simulink model "Traj"  (R2024b)
settings: Solver=VariableStepAuto  StartTime=0.0  StopTime=40  RelTol=1e-3
values from neighbouring files (symbols this model uses):
  K = lqr(A, B, Q, R)    [lq.m]    (also in lqr.m = lqr(A,B,Q,R))
  L = 0.4    [lq.m]    (also in lqr.m = 0.2)
  P = double(P)    [lq.m]    (also in lqr.m)
  theta0 = double(theta0)    [lq.m]    (also in lqr.m)
  theta_ref = double(theta_ref(:))    [lq.m]    (also in lqr.m)
  Ts_ref = double(Ts_ref)    [lq.m]    (also in lqr.m)
  vd_ref = double(vd_ref(:))    [lq.m]    (also in lqr.m)
  wd_ref = double(wd_ref(:))    [lq.m]    (also in lqr.m)
  x0 = double(x0)    [lq.m]    (also in lqr.m)
  y0 = double(y0)    [lq.m]    (also in lqr.m)
libraries: eeGeneralControl x2, slpidlib x2
settings Model: Creator=mwali  LastModifiedBy=mwali
settings ConfigComp: CovBoundaryAbsTol=1.0e-5

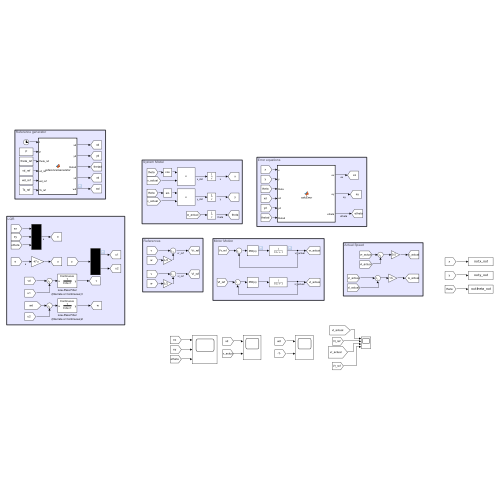
[thumbnail: Simulink's stored preview of the top-level diagram]
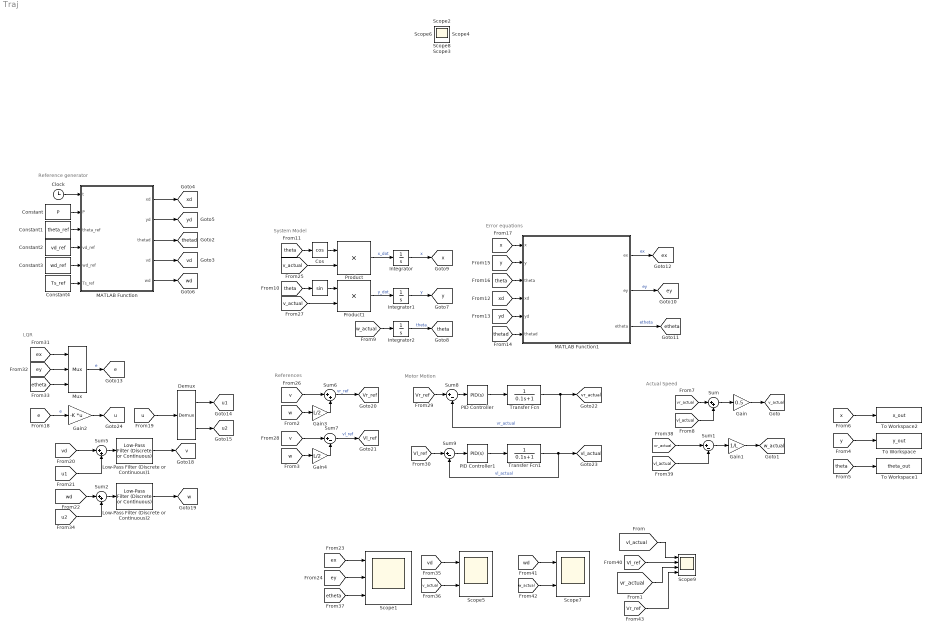
== system Traj ==
  note: Actual Speed
  note: Motor Motion
  note: References
  note: LQR
  note: Error equations
  note: System Model
  note: Reference generator
  " " : Trigonometry
  Clock : Clock
  Constant : Constant  Value=P
  Constant1 : Constant  Value=theta_ref
  Constant2 : Constant  Value=vd_ref
  Constant3 : Constant  Value=wd_ref
  Constant4 : Constant  Value=Ts_ref
  Cos : Trigonometry  Operator=cos
  Demux : Demux  Outputs=2
  Gain : Gain  Gain=0.5
  Gain1 : Gain  Gain=1/L
  Gain2 : Gain  Gain=-K  Multiplication=Matrix(K*u)
  Gain3 : Gain  Gain=L/2
  Gain4 : Gain  Gain=L/2
  Integrator : Integrator  InitialCondition=x0
  Integrator1 : Integrator  InitialCondition=y0
  Integrator2 : Integrator  InitialCondition=theta0
  Low-Pass Filter (Discrete or Continuous)1 : eeGeneralControl/Low-Pass Filter (Discrete or Continuous)  K=1  T=0.6  B=inf  A=-inf  init_option=Inherited from block input  x0=0  Ts=0
  Low-Pass Filter (Discrete or Continuous)2 : eeGeneralControl/Low-Pass Filter (Discrete or Continuous)  K=1  T=0.6  B=inf  A=-inf  init_option=Inherited from block input  x0=0  Ts=0
  MATLAB Function : MATLAB Function  TreatAsAtomicUnit=on
  MATLAB Function1 : MATLAB Function  TreatAsAtomicUnit=on
  Mux : Mux  Inputs=3
  PID Controller : slpidlib/PID Controller  Controller=PID  Form=Parallel  TimeDomain=Continuous-time  UseExternalTs=off  SampleTime=-1  IntegratorMethod=Forward Euler  FilterMethod=Forward Euler  ControllerParametersSource=internal  P=0.9  I=0.04  UseKiTs=off  D=1  UseExternalDerivativeSource=off  N=100  UseFilter=on  TunerSelectOption=Transfer Function Based (PID Tuner App)  InitialConditionSource=internal  InitialConditionForIntegrator=0  InitialConditionForFilter=0  DifferentiatorICPrevScaledInput=0  ExternalReset=none  TrackingMode=off  Kt=1  LimitOutput=off  SatLimitsSource=internal  UpperSaturationLimit=0.5  LowerSaturationLimit=0  LinearizeAsGain=on  AntiWindupMode=clamping  Kb=1  LimitIntegrator=off  UpperIntegratorSaturationLimit=inf  LowerIntegratorSaturationLimit=-inf  POutMin=[]  POutMax=[]  IOutMin=[]  IOutMax=[]  DOutMin=[]  DOutMax=[]  NOutMin=[]  NOutMax=[]  SumOutMin=[]  SumOutMax=[]  SaturationOutMin=[]  SaturationOutMax=[]  PParamMin=[]  PParamMax=[]  IParamMin=[]  IParamMax=[]  DParamMin=[]  DParamMax=[]  NParamMin=[]  NParamMax=[]  KbParamMin=[]  KbParamMax=[]  KtParamMin=[]  KtParamMax=[]  KbOutMin=[]  KbOutMax=[]  KtOutMin=[]  KtOutMax=[]  IntegratorOutMin=[]  IntegratorOutMax=[]  FilterOutMin=[]  FilterOutMax=[]  SumI1OutMin=[]  SumI1OutMax=[]  SumI2OutMin=[]  SumI2OutMax=[]  SumI3OutMin=[]  SumI3OutMax=[]  SumI4OutMin=[]  SumI4OutMax=[]  SumDOutMin=[]  SumDOutMax=[]  DifferentiatorOutMin=[]  DifferentiatorOutMax=[]  FilterDiffOutCoefMin=[]  FilterDiffOutCoefMax=[]  ReciprocalOutMin=[]  ReciprocalOutMax=[]  SumDenOutMin=[]  SumDenOutMax=[]  SumNumOutMin=[]  SumNumOutMax=[]  DivideOutMin=[]  DivideOutMax=[]  UdiffTsProdOutMin=[]  UdiffTsProdOutMax=[]  NTsProdOutMin=[]  NTsProdOutMax=[]  UintegralTsProdOutMin=[]  UintegralTsProdOutMax=[]  UngainTsProdOutMin=[]  UngainTsProdOutMax=[]  ClampingZeroOutDataTypeStr=Inherit: Inherit via back propagation  ClampingZeroOutMin=[]  ClampingZeroOutMax=[]  FilterDenConstantOutDataTypeStr=Inherit: Inherit via back propagation  FilterDenConstantOutMin=[]  FilterDenConstantOutMax=[]  PCopyOutDataTypeStr=Inherit: Inherit via back propagation  PCopyOutMin=[]  PCopyOutMax=[]  NCopyOutDataTypeStr=Inherit: Inherit via back propagation  NCopyOutMin=[]  NCopyOutMax=[]  IntegratorContinuousStateAttributes=''  IntegratorStateMustResolveToSignalObject=off  IntegratorRTWStateStorageClass=Auto  FilterContinuousStateAttributes=''  FilterStateMustResolveToSignalObject=off  FilterRTWStateStorageClass=Auto  ParallelPVariant=InternalParameters  IdealPVariant=Disabled  IVariant=InternalParameters  DVariant=InternalParameters  IntegratorVariant=Continuous  SatVariant=Disabled  AWVariant=Passthrough  PCopyVariant=Disabled  TRVariant=Disabled  FdbkBlocksVariant=Forward  IdealPFdbkVariant=Disabled  SatFdbkVariant=Disabled  DerivativeFilterVariant=ContFilter  NVariant=InternalParameters  NCopyVariant=Disabled  FilterICVariant=InternalICsFilter  IntegratorICVariant=InternalICs  ExternalResetVariant=Disabled  TRSumVariant=Passthrough  SumFdbkVariant=Disabled  SumVariant=Sum_PID  TsampFilterVariant=InternalTs  TsampNgainVariant=Passthrough  TsampIntegralVariant=Disabled_SignalSpec  ExternalSaturationOutDataTypeStr=Inherit: Same as second input  DerivativeSourceVariant=ErrorSignal  PreIntVariant=InternalPreInt
  PID Controller1 : slpidlib/PID Controller  Controller=PID  Form=Parallel  TimeDomain=Continuous-time  UseExternalTs=off  SampleTime=-1  IntegratorMethod=Forward Euler  FilterMethod=Forward Euler  ControllerParametersSource=internal  P=0.9  I=0.04  UseKiTs=off  D=1  UseExternalDerivativeSource=off  N=100  UseFilter=on  TunerSelectOption=Transfer Function Based (PID Tuner App)  InitialConditionSource=internal  InitialConditionForIntegrator=0  InitialConditionForFilter=0  DifferentiatorICPrevScaledInput=0  ExternalReset=none  TrackingMode=off  Kt=1  LimitOutput=off  SatLimitsSource=internal  UpperSaturationLimit=0.5  LowerSaturationLimit=0  LinearizeAsGain=on  AntiWindupMode=clamping  Kb=1  LimitIntegrator=off  UpperIntegratorSaturationLimit=inf  LowerIntegratorSaturationLimit=-inf  POutMin=[]  POutMax=[]  IOutMin=[]  IOutMax=[]  DOutMin=[]  DOutMax=[]  NOutMin=[]  NOutMax=[]  SumOutMin=[]  SumOutMax=[]  SaturationOutMin=[]  SaturationOutMax=[]  PParamMin=[]  PParamMax=[]  IParamMin=[]  IParamMax=[]  DParamMin=[]  DParamMax=[]  NParamMin=[]  NParamMax=[]  KbParamMin=[]  KbParamMax=[]  KtParamMin=[]  KtParamMax=[]  KbOutMin=[]  KbOutMax=[]  KtOutMin=[]  KtOutMax=[]  IntegratorOutMin=[]  IntegratorOutMax=[]  FilterOutMin=[]  FilterOutMax=[]  SumI1OutMin=[]  SumI1OutMax=[]  SumI2OutMin=[]  SumI2OutMax=[]  SumI3OutMin=[]  SumI3OutMax=[]  SumI4OutMin=[]  SumI4OutMax=[]  SumDOutMin=[]  SumDOutMax=[]  DifferentiatorOutMin=[]  DifferentiatorOutMax=[]  FilterDiffOutCoefMin=[]  FilterDiffOutCoefMax=[]  ReciprocalOutMin=[]  ReciprocalOutMax=[]  SumDenOutMin=[]  SumDenOutMax=[]  SumNumOutMin=[]  SumNumOutMax=[]  DivideOutMin=[]  DivideOutMax=[]  UdiffTsProdOutMin=[]  UdiffTsProdOutMax=[]  NTsProdOutMin=[]  NTsProdOutMax=[]  UintegralTsProdOutMin=[]  UintegralTsProdOutMax=[]  UngainTsProdOutMin=[]  UngainTsProdOutMax=[]  ClampingZeroOutDataTypeStr=Inherit: Inherit via back propagation  ClampingZeroOutMin=[]  ClampingZeroOutMax=[]  FilterDenConstantOutDataTypeStr=Inherit: Inherit via back propagation  FilterDenConstantOutMin=[]  FilterDenConstantOutMax=[]  PCopyOutDataTypeStr=Inherit: Inherit via back propagation  PCopyOutMin=[]  PCopyOutMax=[]  NCopyOutDataTypeStr=Inherit: Inherit via back propagation  NCopyOutMin=[]  NCopyOutMax=[]  IntegratorContinuousStateAttributes=''  IntegratorStateMustResolveToSignalObject=off  IntegratorRTWStateStorageClass=Auto  FilterContinuousStateAttributes=''  FilterStateMustResolveToSignalObject=off  FilterRTWStateStorageClass=Auto  ParallelPVariant=InternalParameters  IdealPVariant=Disabled  IVariant=InternalParameters  DVariant=InternalParameters  IntegratorVariant=Continuous  SatVariant=Disabled  AWVariant=Passthrough  PCopyVariant=Disabled  TRVariant=Disabled  FdbkBlocksVariant=Forward  IdealPFdbkVariant=Disabled  SatFdbkVariant=Disabled  DerivativeFilterVariant=ContFilter  NVariant=InternalParameters  NCopyVariant=Disabled  FilterICVariant=InternalICsFilter  IntegratorICVariant=InternalICs  ExternalResetVariant=Disabled  TRSumVariant=Passthrough  SumFdbkVariant=Disabled  SumVariant=Sum_PID  TsampFilterVariant=InternalTs  TsampNgainVariant=Passthrough  TsampIntegralVariant=Disabled_SignalSpec  ExternalSaturationOutDataTypeStr=Inherit: Same as second input  DerivativeSourceVariant=ErrorSignal  PreIntVariant=InternalPreInt
  Product : Product
  Product1 : Product
  Scope1 : Scope  NumInputPorts=3
  Scope5 : Scope  NumInputPorts=2
  Scope7 : Scope  NumInputPorts=2
  Scope9 : Scope  NumInputPorts=4
  Sum{,2,5..6} (4 alike) : Sum  Inputs=|++
  Sum{1,7..9} (4 alike) : Sum  Inputs=|+-
  To Workspace : ToWorkspace  VariableName=y_out  SampleTime=-1
  To Workspace1 : ToWorkspace  VariableName=theta_out  SampleTime=-1
  To Workspace2 : ToWorkspace  VariableName=x_out  SampleTime=-1
  Transfer Fcn : TransferFcn  Denominator=[0.1 1]
  Transfer Fcn1 : TransferFcn  Denominator=[0.1 1]
  Scope{,2..4,6,8} (6 alike) : Scope
  tag scope: Vl_ref=global, Vr_ref=global, e=global, etheta=global, ex=global, ey=global, theta=global, thetad=global, u1=global, u2=global, u=global, v=global, v_actual=global, vd=global, vl_actual=global, vr_actual=global, w=global, w_actual=global, wd=global, x=global, xd=global, y=global, yd=global
  wires:
  [y] -> To Workspace/1
  [theta] -> To Workspace1/1
  [x] -> To Workspace2/1
  [vd] -> Scope5/1
  [v_actual] -> Scope5/2
  [wd] -> Scope7/1
  [w_actual] -> Scope7/2
  [ex] -> Scope1/1
  [ey] -> Scope1/2
  [etheta] -> Scope1/3
  [vl_actual] -> Scope9/1
  [vr_actual] -> Scope9/3
  Constant/1 -> MATLAB Function/2(P)
  Constant2/1 -> MATLAB Function/4(vd_ref)
  Clock/1 -> MATLAB Function/1(t)
  MATLAB Function/4(vd) -> [vd]
  Constant1/1 -> MATLAB Function/3(theta_ref)
  MATLAB Function/5(wd) -> [wd]
  MATLAB Function/3(thetad) -> [thetad]
  Constant4/1 -> MATLAB Function/6(Ts_ref)
  MATLAB Function/2(yd) -> [yd]
  MATLAB Function/1(xd) -> [xd]
  Constant3/1 -> MATLAB Function/5(wd_ref)
  [theta] -> " "/1
  " "/1 -> Product1/1
  Integrator/1 -> [x]  "x"
  Cos/1 -> Product/1
  Integrator2/1 -> [theta]  "theta"
  Product1/1 -> Integrator1/1  "y_dot"
  [w_actual] -> Integrator2/1
  Product/1 -> Integrator/1  "x_dot"
  [v_actual] -> Product/2
  [v_actual] -> Product1/2
  Integrator1/1 -> [y]  "y"
  [theta] -> Cos/1
  MATLAB Function1/3(etheta) -> [etheta]  "etheta"
  MATLAB Function1/2(ey) -> [ey]  "ey"
  MATLAB Function1/1(ex) -> [ex]  "ex"
  [theta] -> MATLAB Function1/3(theta)
  [y] -> MATLAB Function1/2(y)
  [x] -> MATLAB Function1/1(x)
  [xd] -> MATLAB Function1/4(xd)
  [yd] -> MATLAB Function1/5(yd)
  [thetad] -> MATLAB Function1/6(thetad)
  [e] -> Gain2/1  "e"
  [u1] -> Sum5/2
  Low-Pass Filter (Discrete or Continuous)1/1 -> [v]
  [ey] -> Mux/2
  [ex] -> Mux/1
  [wd] -> Sum2/1
  Mux/1 -> [e]  "e"
  [etheta] -> Mux/3
  Demux/1 -> [u1]
  [u2] -> Sum2/2
  Gain2/1 -> [u]
  Sum2/1 -> Low-Pass Filter (Discrete or Continuous)2/1
  [vd] -> Sum5/1
  Demux/2 -> [u2]
  Low-Pass Filter (Discrete or Continuous)2/1 -> [w]
  [u] -> Demux/1
  Sum5/1 -> Low-Pass Filter (Discrete or Continuous)1/1
  [v] -> Sum7/1
  [w] -> Gain4/1
  Sum6/1 -> [Vr_ref]  "vr_ref"
  Gain4/1 -> Sum7/2
  [w] -> Gain3/1
  [v] -> Sum6/1
  Sum7/1 -> [Vl_ref]  "vl_ref"
  Gain3/1 -> Sum6/2
  Sum8/1 -> PID Controller/1
  Transfer Fcn/1 -> [vr_actual], Sum8/2  "vr_actual"
  [Vr_ref] -> Sum8/1
  [Vl_ref] -> Sum9/1
  PID Controller1/1 -> Transfer Fcn1/1
  Sum9/1 -> PID Controller1/1
  Transfer Fcn1/1 -> [vl_actual], Sum9/2  "vl_actual"
  PID Controller/1 -> Transfer Fcn/1
  Gain1/1 -> [w_actual]
  [vr_actual] -> Sum/1
  Gain/1 -> [v_actual]
  Sum/1 -> Gain/1
  [vr_actual] -> Sum1/1
  [vl_actual] -> Sum/2
  [vl_actual] -> Sum1/2
  Sum1/1 -> Gain1/1
  [Vl_ref] -> Scope9/2
  [Vr_ref] -> Scope9/4

== matlab function Traj/MATLAB Function1 ==
  data: x input; ex output; y input; theta input; xd input; yd input; thetad input; ey output; etheta output
function [ex, ey, etheta] = calcError(x, y, theta, xd, yd, thetad)

dx = x - xd;
dy = y - yd;

ex =  cos(thetad)*dx + sin(thetad)*dy;
ey = -sin(thetad)*dx + cos(thetad)*dy;

etheta = atan2(sin(theta - thetad), cos(theta - thetad));

== matlab function Traj/MATLAB Function ==
  data: t input; P input; theta_ref input; vd_ref input; wd_ref input; Ts_ref input; xd output; yd output; thetad output; vd output; wd output
function [xd, yd, thetad, vd, wd] = referenceGenerator(t, P, theta_ref, vd_ref, wd_ref, Ts_ref)

idx = round(t / Ts_ref) + 1;

if idx < 1
    idx = 1;
elseif idx > size(P,1)
    idx = size(P,1);
end

xd     = P(idx,1);
yd     = P(idx,2);
thetad = theta_ref(idx,1);
vd     = vd_ref(idx,1);
wd     = wd_ref(idx,1);
